simulink model "Atmos_VarAeroBlock"  (R2016b)
settings: Solver=VariableStepAuto  StartTime=0.0  StopTime=10.0  RelTol=1e-3
undefined symbols (not defined in the file or in its folder): Env, HDBK, Light, MIL
libraries: aerolibwind2 x2, aerolibatmos2 x1
settings Model: Creator=rega0051  LastModifiedBy=rega0051
settings DataIOCC: SaveOutput=off  SignalLogging=off  DSMLogging=off  SaveTime=off

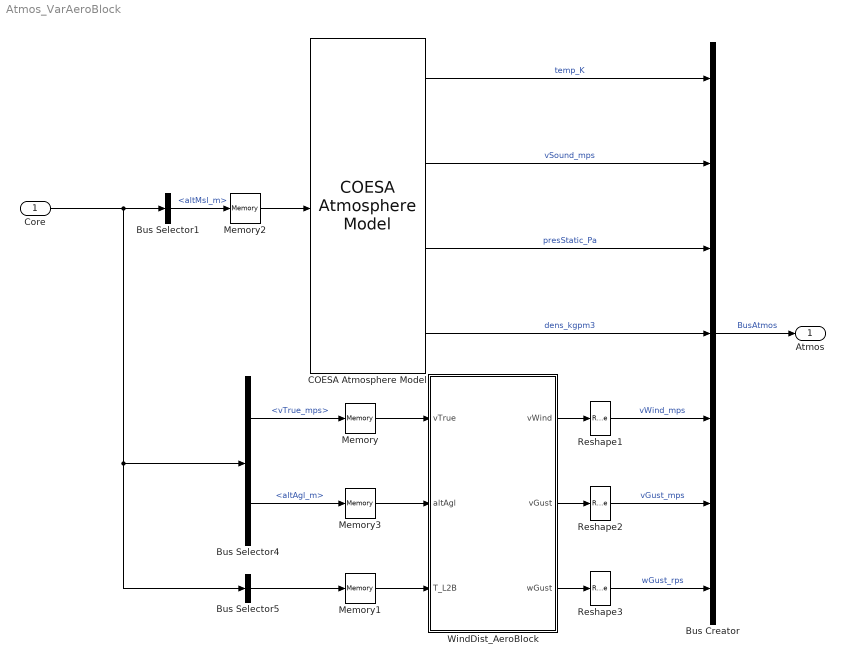
== system Atmos_VarAeroBlock ==
  Core : Inport  OutDataTypeStr=Bus: BusCore
      settings: AttributesFormatString=%<OutDataTypeStr>
  Bus Creator : BusCreator  Inputs=7  OutDataTypeStr=Bus: BusAtmos
      settings: AttributesFormatString=%<OutDataTypeStr>
  Bus Selector1 : BusSelector  OutputSignals=BusAux.BusNav.altMsl_m
  Bus Selector4 : BusSelector  OutputSignals=BusAux.BusFlow.vTrue_mps,BusAux.BusNav.altAgl_m
  Bus Selector5 : BusSelector  OutputSignals=BusEom.T_L2B  OutputAsBus=on
  COESA Atmosphere Model : aerolibatmos2/COESA Atmosphere Model  units=Metric (MKS)  spec=1976 COESA-extended U.S. Standard Atmosphere  model=Profile  profile_var=High temperature  profile_percent=1%  profile_alt=5 km (16404 ft)  envelope_var=High temperature  envelope_percent=1%  action=Warning
  Memory{,1..3} (4 alike) : Memory
  Reshape1 : Reshape  OutputDimensionality=Column vector (2-D)  OutputDimensions=[3,1]
  Reshape2 : Reshape  OutputDimensionality=Column vector (2-D)  OutputDimensions=[3,1]
  Reshape3 : Reshape  OutputDimensionality=Column vector (2-D)  OutputDimensions=[3,1]
  WindDist_AeroBlock : Subsystem
  Atmos : Outport  OutDataTypeStr=Bus: BusAtmos
      settings: AttributesFormatString=%<OutDataTypeStr>
  wires:
  Reshape3/1 -> Bus Creator/7  "wGust_rps"
  Reshape2/1 -> Bus Creator/6  "vGust_mps"
  Reshape1/1 -> Bus Creator/5  "vWind_mps"
  WindDist_AeroBlock/1(vWind) -> Reshape1/1
  WindDist_AeroBlock/3(wGust) -> Reshape3/1
  WindDist_AeroBlock/2(vGust) -> Reshape2/1
  Bus Selector1/1 -> Memory2/1  "<altMsl_m>"
  Bus Selector5/1 -> Memory1/1
  Bus Selector4/1 -> Memory/1  "<vTrue_mps>"
  COESA Atmosphere Model/4 -> Bus Creator/4  "dens_kgpm3"
  COESA Atmosphere Model/3 -> Bus Creator/3  "presStatic_Pa"
  COESA Atmosphere Model/2 -> Bus Creator/2  "vSound_mps"
  COESA Atmosphere Model/1 -> Bus Creator/1  "temp_K"
  Core/1 -> Bus Selector1/1, Bus Selector4/1, Bus Selector5/1
  Bus Creator/1 -> Atmos/1  "BusAtmos"
  Bus Selector4/2 -> Memory3/1  "<altAgl_m>"
  Memory/1 -> WindDist_AeroBlock/1(vTrue)
  Memory2/1 -> COESA Atmosphere Model/1
  Memory3/1 -> WindDist_AeroBlock/2(altAgl)
  Memory1/1 -> WindDist_AeroBlock/3(T_L2B)

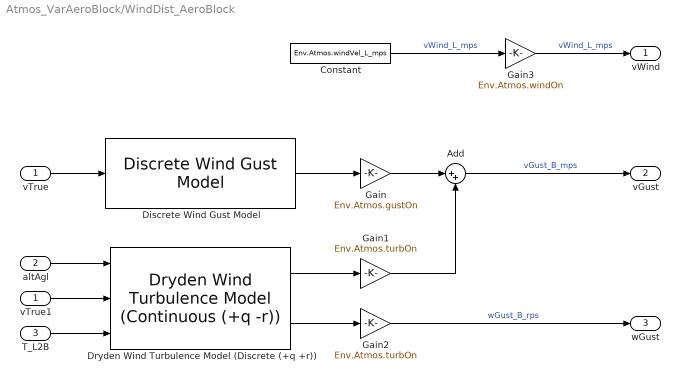
== system Atmos_VarAeroBlock/WindDist_AeroBlock ==
  vTrue : Inport
  altAgl : Inport  Port=2
  T_L2B : Inport  Port=3
  Add : Sum  Inputs=|++
  Constant : Constant  Value=Env.Atmos.windVel_L_mps
      settings: AttributesFormatString=%<Value>
  Discrete Wind Gust Model : aerolibwind2/Discrete Wind Gust Model  units=Metric (MKS)  Gx=on  Gy=on  Gz=on  t_0=Env.Atmos.gustTimeStart_s  d_m=Env.Atmos.gustLen_m  v_m=Env.Atmos.gustVelMag_B_mps
  Dryden Wind Turbulence Model (Discrete (+q +r)) : aerolibwind2/Dryden Wind Turbulence Model  (Continuous (+q -r))  units=Metric (MKS)  spec=MIL-HDBK-1797B  model=Discrete Dryden (+q +r)  W20=Env.Atmos.windVelMag_mps  Wdeg=Env.Atmos.windVelDir_deg  TurbProb=10^-2 - Light  L_high=762  Wingspan=Env.Atmos.turbSpan_m  ts=Env.Atmos.turbTimeSample_s  Seed=Env.Atmos.turbSeed  T_on=on
  Gain : Gain  Gain=Env.Atmos.gustOn
      settings: AttributesFormatString=%<Gain>
  Gain1 : Gain  Gain=Env.Atmos.turbOn
      settings: AttributesFormatString=%<Gain>
  Gain2 : Gain  Gain=Env.Atmos.turbOn
      settings: AttributesFormatString=%<Gain>
  Gain3 : Gain  Gain=Env.Atmos.windOn
      settings: AttributesFormatString=%<Gain>
  vTrue1 : InportShadow
  vWind : Outport
  vGust : Outport  Port=2
  wGust : Outport  Port=3
  wires:
  Gain2/1 -> wGust/1  "wGust_B_rps"
  Add/1 -> vGust/1  "vGust_B_mps"
  vTrue1/1 -> Dryden Wind Turbulence Model (Discrete (+q +r))/2
  altAgl/1 -> Dryden Wind Turbulence Model (Discrete (+q +r))/1
  T_L2B/1 -> Dryden Wind Turbulence Model (Discrete (+q +r))/3
  Dryden Wind Turbulence Model (Discrete (+q +r))/2 -> Gain2/1
  Gain1/1 -> Add/2
  Gain/1 -> Add/1
  Gain3/1 -> vWind/1  "vWind_L_mps"
  Dryden Wind Turbulence Model (Discrete (+q +r))/1 -> Gain1/1
  Discrete Wind Gust Model/1 -> Gain/1
  Constant/1 -> Gain3/1  "vWind_L_mps"
  vTrue/1 -> Discrete Wind Gust Model/1
